simulink model "Controlled_3ph_FullWave"  (R2021a)
settings: Solver=VariableStepAuto  StartTime=0.0  StopTime=0.8  MaxStep=1e-6  RelTol=1e-3
libraries: spsThyristorLib x6, spsACVoltageSourceLib x3, spsControlledCurrentSourceLib x1, spsGroundLib x1, spsMeanLib x1, spsVoltageMeasurementLib x1, spspowerguiLib x1
settings Model: Creator=Shashwat M.A  LastModifiedBy=Shashwat M.A

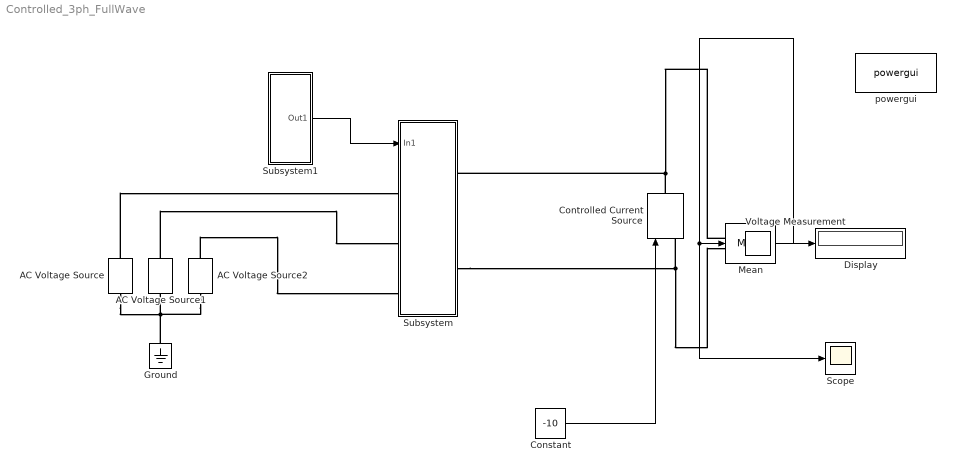
== system Controlled_3ph_FullWave ==
  AC Voltage Source : spsACVoltageSourceLib/AC Voltage Source  Amplitude=325  Phase=0  Frequency=50  SampleTime=0  Measurements=None  BusType=swing  Pref=10e3  Qref=0  Qmin=-inf  Qmax=+inf
  AC Voltage Source1 : spsACVoltageSourceLib/AC Voltage Source  Amplitude=325  Phase=-120  Frequency=50  SampleTime=0  Measurements=None  BusType=swing  Pref=10e3  Qref=0  Qmin=-inf  Qmax=+inf
  AC Voltage Source2 : spsACVoltageSourceLib/AC Voltage Source  Amplitude=325  Phase=-240  Frequency=50  SampleTime=0  Measurements=None  BusType=swing  Pref=10e3  Qref=0  Qmin=-inf  Qmax=+inf
  Constant : Constant  Value=-10
  Controlled Current Source : spsControlledCurrentSourceLib/Controlled Current Source  Initialize=on  Source_Type=AC  Amplitude=0  Phase=0  Frequency=0  Measurements=None
  Display : Display
  Ground : spsGroundLib/Ground  LConnTagsString=a
  Mean : spsMeanLib/Mean  Freq=50*6  Vinit=0  Ts=0
  Scope : Scope
  Subsystem : Subsystem
  Subsystem1 : Subsystem
  Voltage Measurement : spsVoltageMeasurementLib/Voltage Measurement  PhasorSimulation=off  OutputType=Complex  PSBequivalent=0
  powergui : spspowerguiLib/powergui  Priority=1  SimulationMode=Continuous  SampleTime=50e-6  frequency=60  Iterations=50  frequencyindice=50  Pbase=100e6  ErrMax=1e-4  UnitsV=kV  UnitsW=MW  buscounter=0  FunctionMessages=off  echomessages=off  EnableUseOfTLC=off  CurrentSourceSwitches=off  DisableSnubberDevices=off  DisableRonSwitches=off  DisableVfSwitches=off  DisplayEquations=off  AutomaticDiscreteSolvers=off  SolverType=Tustin/Backward Euler (TBE)  Interpol=off  ExternalGateDelay=off  methode=off  Ts=100  x0status=blocks  SPID=on  SwTol=0  HookPort=off  NonlinearTolerance=1e-4  nMaxIteration=100  ContinueOnMaxIteration=off  RestoreLinks=warning  ResistiveCurrentMeasurement=off  Frange=[0:2:500]  Ylog=off  Xlog=on  ShowGrid=off  save=off  variable=ZData  structure=0  ZoomFFT=off  StartTime=0.0  cycles=1  DisplayStyle=1  fundamental=60  FreqAxis=off  MaxFrequency=1000  frequencyindicesteady=1  RmsSteady=1  display=off
  wires:
  Voltage Measurement/1 -> Scope/1, Mean/1
  Mean/1 -> Display/1
  Constant/1 -> Controlled Current Source/1
  Subsystem1/1(Out1) -> Subsystem/1(In1)
  connections:
  AC Voltage Source/LConn1 -- Ground/LConn1 -- AC Voltage Source2/LConn1 -- AC Voltage Source1/LConn1
  Subsystem/RConn2 -- Controlled Current Source/LConn1 -- Voltage Measurement/LConn2
  Controlled Current Source/RConn1 -- Voltage Measurement/LConn1 -- Subsystem/RConn1
  AC Voltage Source/RConn1 -- Subsystem/LConn1
  AC Voltage Source1/RConn1 -- Subsystem/LConn2
  AC Voltage Source2/RConn1 -- Subsystem/LConn3

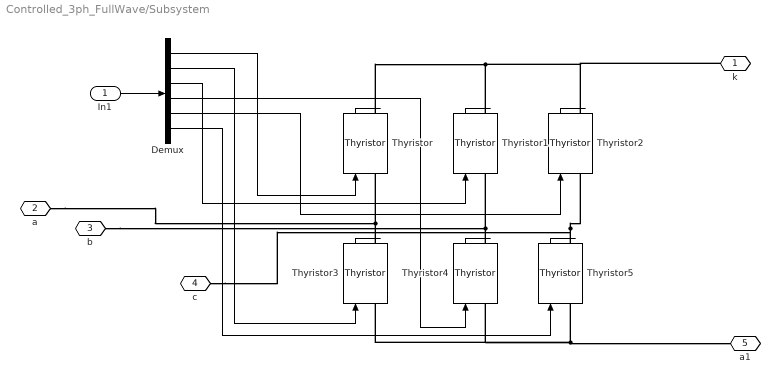
== system Controlled_3ph_FullWave/Subsystem ==
  In1 : Inport
  Demux : Demux  Outputs=6
  Thyristor{,1..5} (6 alike) : spsThyristorLib/Thyristor  Ron=0.001  Lon=0  Vf=0.8  IC=0  Rs=500  Cs=250e-9  Measurements=on
  k : PMIOPort  Side=Right
  a : PMIOPort  Port=2  Side=Left
  b : PMIOPort  Port=3  Side=Left
  c : PMIOPort  Port=4  Side=Left
  a1 : PMIOPort  Port=5  Side=Right
  wires:
  Thyristor3/1 -> ?
  Thyristor1/1 -> ?
  Demux/4 -> Thyristor4/1
  Thyristor5/1 -> ?
  Demux/3 -> Thyristor1/1
  Demux/6 -> Thyristor5/1
  Thyristor/1 -> ?
  Demux/1 -> Thyristor/1
  Thyristor2/1 -> ?
  Demux/2 -> Thyristor3/1
  Demux/5 -> Thyristor2/1
  Thyristor4/1 -> ?
  In1/1 -> Demux/1
  connections:
  Thyristor3/LConn1 -- Thyristor4/LConn1 -- a1/RConn1 -- Thyristor5/LConn1
  Thyristor5/RConn1 -- Thyristor2/LConn1 -- c/RConn1
  k/RConn1 -- Thyristor2/RConn1 -- Thyristor1/RConn1 -- Thyristor/RConn1
  Thyristor3/RConn1 -- Thyristor/LConn1 -- a/RConn1
  Thyristor4/RConn1 -- Thyristor1/LConn1 -- b/RConn1

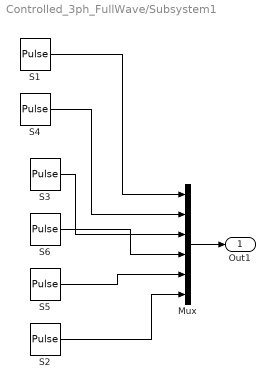
== system Controlled_3ph_FullWave/Subsystem1 ==
  Mux : Mux  Inputs=6
  S1 : DiscretePulseGenerator  PulseType=Time based  Period=0.02  PulseWidth=1/3*100
  S2 : DiscretePulseGenerator  PulseType=Time based  Period=0.02  PulseWidth=1/3*100  PhaseDelay=-60/360*0.02
  S3 : DiscretePulseGenerator  PulseType=Time based  Period=0.02  PulseWidth=1/3*100  PhaseDelay=-120/360*0.02
  S4 : DiscretePulseGenerator  PulseType=Time based  Period=0.02  PulseWidth=1/3*100  PhaseDelay=-180/360*0.02
  S5 : DiscretePulseGenerator  PulseType=Time based  Period=0.02  PulseWidth=1/3*100  PhaseDelay=-240/360*0.02
  S6 : DiscretePulseGenerator  PulseType=Time based  Period=0.02  PulseWidth=1/3*100  PhaseDelay=-300/360*0.02
  Out1 : Outport
  wires:
  S1/1 -> Mux/1
  S4/1 -> Mux/2
  S3/1 -> Mux/3
  S6/1 -> Mux/4
  S5/1 -> Mux/5
  S2/1 -> Mux/6
  Mux/1 -> Out1/1
